simulink model "PID_Controller"  (R2018b)
settings: Solver=ode23s  StartTime=0.0  StopTime=10.0  RelTol=1e-3  AbsTol=AUTO  EnableMultiTasking=on
undefined symbols (not defined in the file or in its folder): Fmatrix, Imatrix
libraries: dspinverses x1
(part 1 of 5)
settings Model: Creator=as01398  LastModifiedBy=jiang
settings SolverCC: MaxConsecutiveMinStep=500
settings DataIOCC: OutputOption=SpecifiedOutputTimes  OutputTimes=[0:0.2:10]
settings OptimizationCC: LifeSpan=inf
settings DebuggingCC: SFUnexpectedBacktrackingDiag=warning  SFNoUnconditionalDefaultTransitionDiag=warning
settings SFSimCC: SimUseLocalCustomCode=off
settings RTWCC: RTWUseLocalCustomCode=off
settings CodeAppCC: StateflowObjectComments=on
settings GRTTargetCC: TargetLangStandard=C89/C90 (ANSI)  GeneratePreprocessorConditionals=Disable all
settings ConfigComp: CovMetricSettings=dw  CovHtmlReporting=on  CovSaveCumulativeToWorkspaceVar=on  CovSaveSingleToWorkspaceVar=on  CovExternalEMLEnable=off

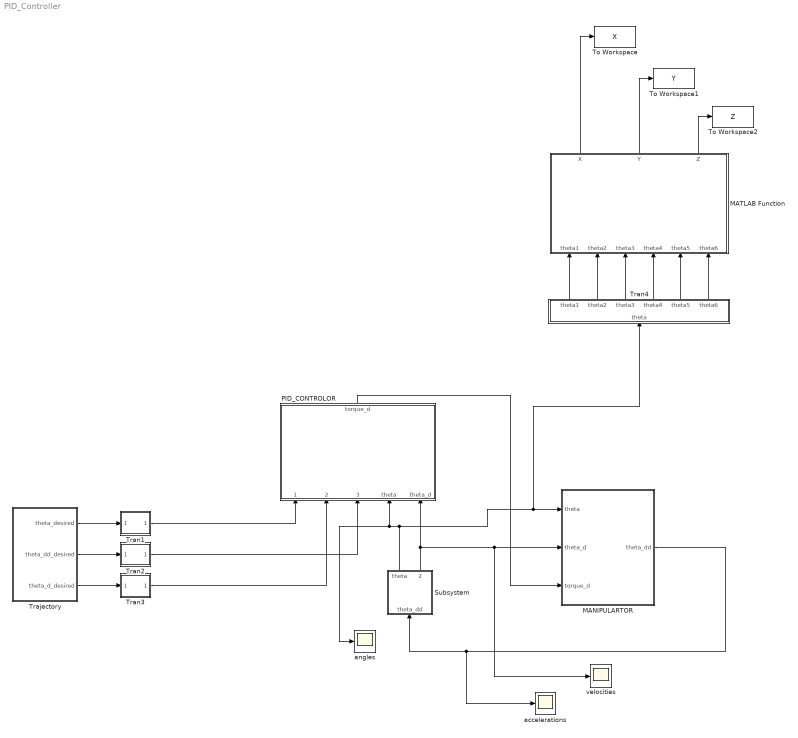
== system PID_Controller ==
  MANIPULARTOR : Subsystem
  MATLAB Function : MATLAB Function  TreatAsAtomicUnit=on
  PID_CONTROLOR : Subsystem
  Subsystem : Subsystem
  To Workspace : ToWorkspace  VariableName=X  SaveFormat=Timeseries  SampleTime=-1
  To Workspace1 : ToWorkspace  VariableName=Y  SaveFormat=Timeseries  SampleTime=-1
  To Workspace2 : ToWorkspace  VariableName=Z  SaveFormat=Timeseries  SampleTime=-1
  Trajectory : Subsystem
  Tran1 : Subsystem
  Tran2 : Subsystem
  Tran3 : Subsystem
  Tran4 : Subsystem
  accelerations : Scope
  angles : Scope
  velocities : Scope
  wires:
  MANIPULARTOR/1(theta_dd) -> accelerations/1, Subsystem/1(theta_dd)
  Subsystem/1(theta) -> PID_CONTROLOR/4(theta), angles/1, Tran4/1(theta), MANIPULARTOR/1(theta)
  Subsystem/2(theta_d) -> PID_CONTROLOR/5(theta_d), velocities/1, MANIPULARTOR/2(theta_d)
  MATLAB Function/1(X) -> To Workspace/1
  MATLAB Function/2(Y) -> To Workspace1/1
  MATLAB Function/3(Z) -> To Workspace2/1
  PID_CONTROLOR/1(torque_d) -> MANIPULARTOR/3(torque_d)
  Trajectory/1(theta_desired) -> Tran1/1(In1)
  Tran1/1(Out2) -> PID_CONTROLOR/1(theta_desired)
  Trajectory/2(theta_dd_desired) -> Tran2/1(In1)
  Tran2/1(Out2) -> PID_CONTROLOR/3(theta_dd_desired)
  Trajectory/3(theta_d_desired) -> Tran3/1(In1)
  Tran3/1(Out2) -> PID_CONTROLOR/2(theta_d_desired)
  Tran4/1(theta1) -> MATLAB Function/1(theta1)
  Tran4/2(theta2) -> MATLAB Function/2(theta2)
  Tran4/3(theta3) -> MATLAB Function/3(theta3)
  Tran4/4(theta4) -> MATLAB Function/4(theta4)
  Tran4/5(theta5) -> MATLAB Function/5(theta5)
  Tran4/6(theta6) -> MATLAB Function/6(theta6)

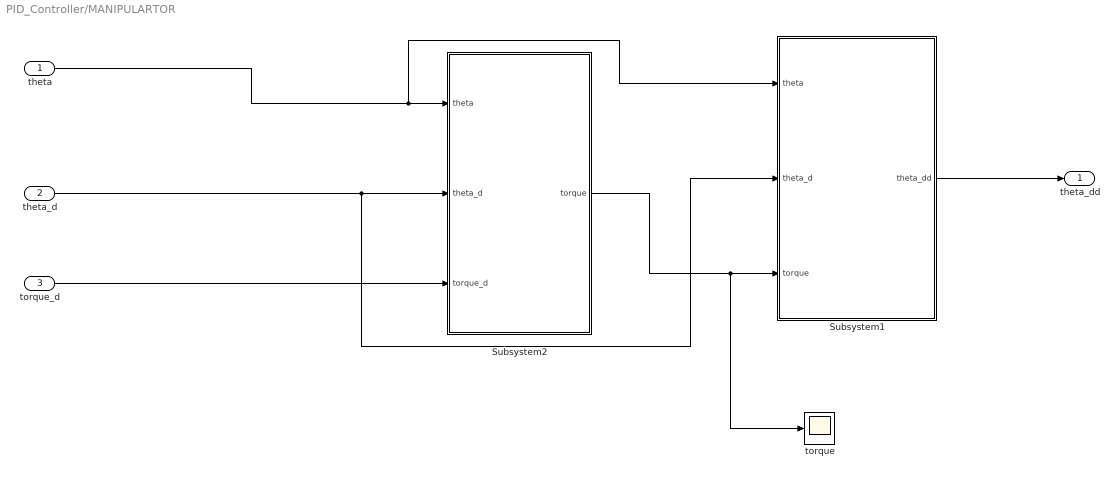
== system PID_Controller/MANIPULARTOR ==
  theta : Inport
  theta_d : Inport  Port=2
  torque_d : Inport  Port=3
  Subsystem1 : Subsystem
  Subsystem2 : Subsystem
  torque : Scope
  theta_dd : Outport
  wires:
  Subsystem1/1(theta_dd) -> theta_dd/1
  torque_d/1 -> Subsystem2/3(torque_d)
  Subsystem2/1(torque) -> torque/1, Subsystem1/3(torque)
  theta/1 -> Subsystem1/1(theta), Subsystem2/1(theta)
  theta_d/1 -> Subsystem1/2(theta_d), Subsystem2/2(theta_d)

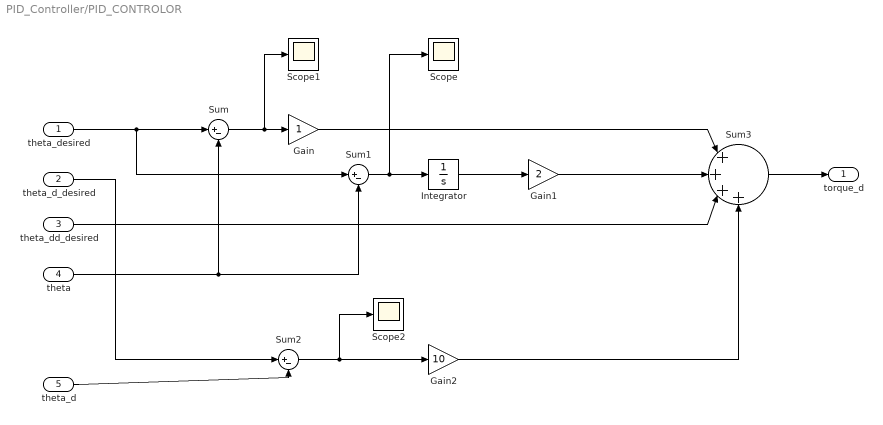
== system PID_Controller/PID_CONTROLOR ==
  theta_desired : Inport
  theta_d_desired : Inport  Port=2
  theta_dd_desired : Inport  Port=3
  theta : Inport  Port=4
  theta_d : Inport  Port=5
  Gain : Gain
  Gain1 : Gain  Gain=2
  Gain2 : Gain  Gain=10
  Integrator : Integrator
  Scope : Scope
  Scope1 : Scope
  Scope2 : Scope
  Sum : Sum  Inputs=|+-
  Sum1 : Sum  Inputs=|+-
  Sum2 : Sum  Inputs=|+-
  Sum3 : Sum  Inputs=|++++
  torque_d : Outport
  wires:
  Sum3/1 -> torque_d/1
  theta_dd_desired/1 -> Sum3/3
  theta_desired/1 -> Sum1/1, Sum/1
  theta/1 -> Sum1/2, Sum/2
  Sum/1 -> Scope1/1, Gain/1
  Sum1/1 -> Integrator/1, Scope/1
  Gain/1 -> Sum3/1
  Gain1/1 -> Sum3/2
  Integrator/1 -> Gain1/1
  Gain2/1 -> Sum3/4
  Sum2/1 -> Scope2/1, Gain2/1
  theta_d_desired/1 -> Sum2/1
  theta_d/1 -> Sum2/2

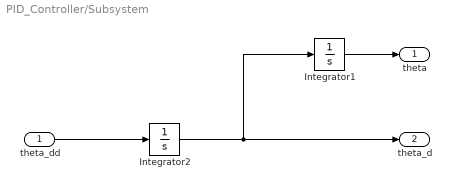
== system PID_Controller/Subsystem ==
  theta_dd : Inport
  Integrator1 : Integrator
  Integrator2 : Integrator
  theta : Outport
  theta_d : Outport  Port=2
  wires:
  theta_dd/1 -> Integrator2/1
  Integrator1/1 -> theta/1
  Integrator2/1 -> theta_d/1, Integrator1/1

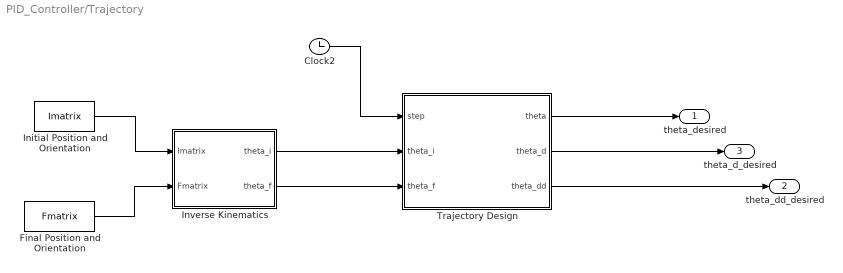
== system PID_Controller/Trajectory ==
  Clock2 : Clock
      settings: Decimation=1000
  Final Position and Orientation : Constant  Value=Fmatrix
  Initial Position and Orientation : Constant  Value=Imatrix
  Inverse Kinematics : MATLAB Function  TreatAsAtomicUnit=on
  Trajectory Design : MATLAB Function  TreatAsAtomicUnit=on
  theta_desired : Outport
  theta_dd_desired : Outport  Port=2
  theta_d_desired : Outport  Port=3
  wires:
  Trajectory Design/3(theta_dd) -> theta_dd_desired/1
  Trajectory Design/2(theta_d) -> theta_d_desired/1
  Trajectory Design/1(theta) -> theta_desired/1
  Inverse Kinematics/2(theta_f) -> Trajectory Design/3(theta_f)
  Inverse Kinematics/1(theta_i) -> Trajectory Design/2(theta_i)
  Final Position and Orientation/1 -> Inverse Kinematics/2(Fmatrix)
  Initial Position and Orientation/1 -> Inverse Kinematics/1(Imatrix)
  Clock2/1 -> Trajectory Design/1(step)

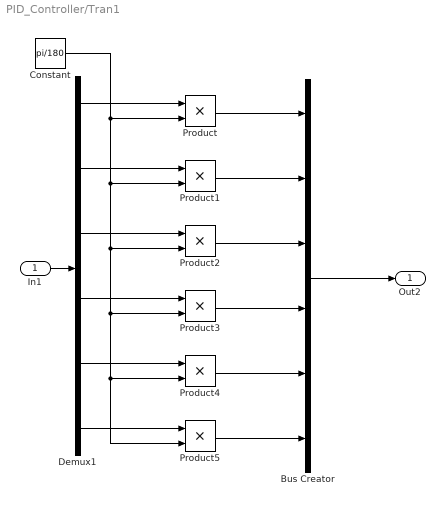
== system PID_Controller/Tran1 ==
  In1 : Inport
  Bus Creator : BusCreator  Inputs=6
  Constant : Constant  Value=pi/180
  Demux1 : Demux  Outputs=6
  Product{,1..5} (6 alike) : Product
  Out2 : Outport
  wires:
  In1/1 -> Demux1/1
  Demux1/1 -> Product/1
  Demux1/2 -> Product1/1
  Demux1/3 -> Product2/1
  Demux1/4 -> Product3/1
  Demux1/5 -> Product4/1
  Demux1/6 -> Product5/1
  Constant/1 -> Product/2, Product1/2, Product2/2, Product3/2, Product5/2, Product4/2
  Product/1 -> Bus Creator/1
  Product1/1 -> Bus Creator/2
  Product2/1 -> Bus Creator/3
  Product3/1 -> Bus Creator/4
  Product4/1 -> Bus Creator/5
  Product5/1 -> Bus Creator/6
  Bus Creator/1 -> Out2/1

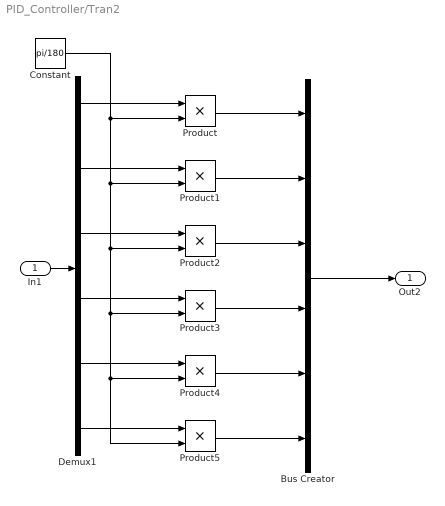
== system PID_Controller/Tran2 ==
  In1 : Inport
  Bus Creator : BusCreator  Inputs=6
  Constant : Constant  Value=pi/180
  Demux1 : Demux  Outputs=6
  Product{,1..5} (6 alike) : Product
  Out2 : Outport
  wires:
  In1/1 -> Demux1/1
  Demux1/1 -> Product/1
  Demux1/2 -> Product1/1
  Demux1/3 -> Product2/1
  Demux1/4 -> Product3/1
  Demux1/5 -> Product4/1
  Demux1/6 -> Product5/1
  Constant/1 -> Product/2, Product1/2, Product2/2, Product3/2, Product5/2, Product4/2
  Product/1 -> Bus Creator/1
  Product1/1 -> Bus Creator/2
  Product2/1 -> Bus Creator/3
  Product3/1 -> Bus Creator/4
  Product4/1 -> Bus Creator/5
  Product5/1 -> Bus Creator/6
  Bus Creator/1 -> Out2/1

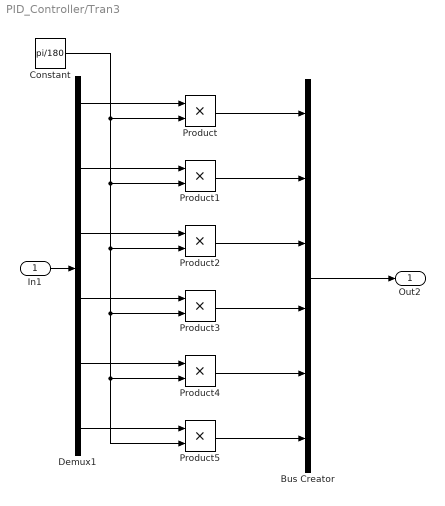
== system PID_Controller/Tran3 ==
  In1 : Inport
  Bus Creator : BusCreator  Inputs=6
  Constant : Constant  Value=pi/180
  Demux1 : Demux  Outputs=6
  Product{,1..5} (6 alike) : Product
  Out2 : Outport
  wires:
  In1/1 -> Demux1/1
  Demux1/1 -> Product/1
  Demux1/2 -> Product1/1
  Demux1/3 -> Product2/1
  Demux1/4 -> Product3/1
  Demux1/5 -> Product4/1
  Demux1/6 -> Product5/1
  Constant/1 -> Product/2, Product1/2, Product2/2, Product3/2, Product5/2, Product4/2
  Product/1 -> Bus Creator/1
  Product1/1 -> Bus Creator/2
  Product2/1 -> Bus Creator/3
  Product3/1 -> Bus Creator/4
  Product4/1 -> Bus Creator/5
  Product5/1 -> Bus Creator/6
  Bus Creator/1 -> Out2/1

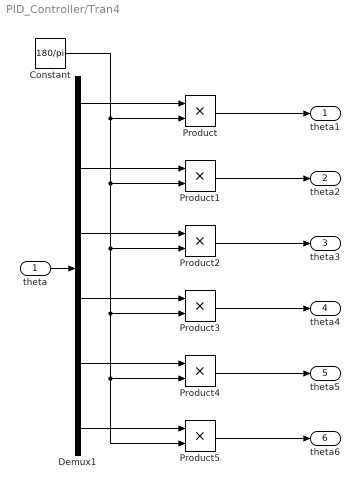
== system PID_Controller/Tran4 ==
  theta : Inport
  Constant : Constant  Value=180/pi
  Demux1 : Demux  Outputs=6
  Product{,1..5} (6 alike) : Product
  theta1 : Outport
  theta2 : Outport  Port=2
  theta3 : Outport  Port=3
  theta4 : Outport  Port=4
  theta5 : Outport  Port=5
  theta6 : Outport  Port=6
  wires:
  theta/1 -> Demux1/1
  Demux1/1 -> Product/1
  Demux1/2 -> Product1/1
  Demux1/3 -> Product2/1
  Demux1/4 -> Product3/1
  Demux1/5 -> Product4/1
  Demux1/6 -> Product5/1
  Constant/1 -> Product/2, Product1/2, Product2/2, Product3/2, Product5/2, Product4/2
  Product/1 -> theta1/1
  Product1/1 -> theta2/1
  Product2/1 -> theta3/1
  Product3/1 -> theta4/1
  Product4/1 -> theta5/1
  Product5/1 -> theta6/1

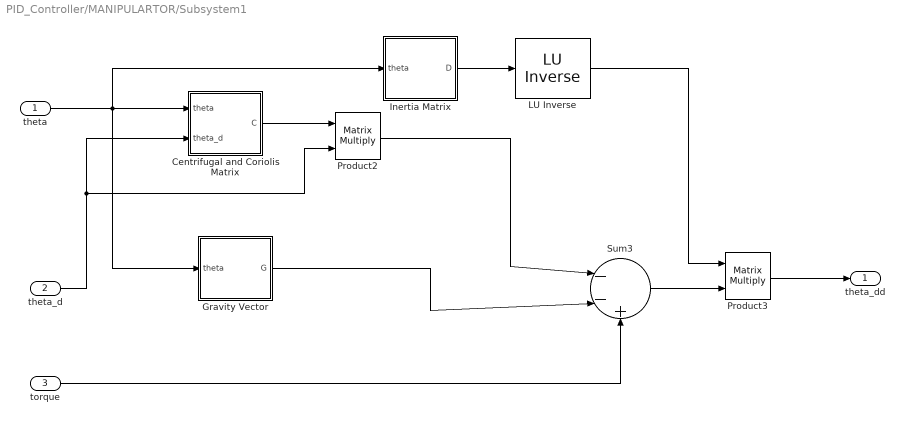
== system PID_Controller/MANIPULARTOR/Subsystem1 ==
  theta : Inport
  theta_d : Inport  Port=2
  torque : Inport  Port=3
  " LU Inverse" : dspinverses/ LU Inverse
      settings: SourceProductName=DSP System Toolbox
  Centrifugal and Coriolis Matrix : Subsystem
  Gravity Vector : Subsystem
  Inertia Matrix : Subsystem
  Product2 : Product  Multiplication=Matrix(*)
  Product3 : Product  Multiplication=Matrix(*)
  Sum3 : Sum  Inputs=|--+
  theta_dd : Outport
  wires:
  Product3/1 -> theta_dd/1
  theta/1 -> Inertia Matrix/1(theta), Gravity Vector/1(theta), Centrifugal and Coriolis Matrix/1(theta)
  theta_d/1 -> Product2/2, Centrifugal and Coriolis Matrix/2(theta_d)
  torque/1 -> Sum3/3
  Gravity Vector/1(G) -> Sum3/2
  Centrifugal and Coriolis Matrix/1(C) -> Product2/1
  Product2/1 -> Sum3/1
  Sum3/1 -> Product3/2
  Inertia Matrix/1(D) -> " LU Inverse"/1
  " LU Inverse"/1 -> Product3/1

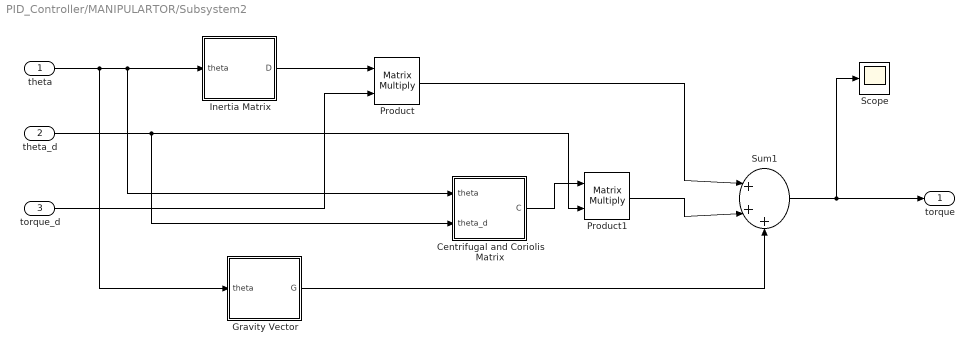
== system PID_Controller/MANIPULARTOR/Subsystem2 ==
  theta : Inport
  theta_d : Inport  Port=2
  torque_d : Inport  Port=3
  Centrifugal and Coriolis Matrix : Subsystem
  Gravity Vector : Subsystem
  Inertia Matrix : Subsystem
  Product : Product  Multiplication=Matrix(*)
  Product1 : Product  Multiplication=Matrix(*)
  Scope : Scope
  Sum1 : Sum  Inputs=|+++
  torque : Outport
  wires:
  theta_d/1 -> Centrifugal and Coriolis Matrix/2(theta_d), Product1/2
  Product/1 -> Sum1/1
  torque_d/1 -> Product/2
  Sum1/1 -> torque/1, Scope/1
  Gravity Vector/1(G) -> Sum1/3
  theta/1 -> Gravity Vector/1(theta), Centrifugal and Coriolis Matrix/1(theta), Inertia Matrix/1(theta)
  Inertia Matrix/1(D) -> Product/1
  Product1/1 -> Sum1/2
  Centrifugal and Coriolis Matrix/1(C) -> Product1/1

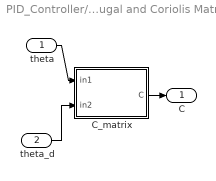
== system PID_Controller/MANIPULARTOR/Subsystem1/Centrifugal and Coriolis Matrix ==
  theta : Inport
  theta_d : Inport  Port=2
  C_matrix : MATLAB Function  TreatAsAtomicUnit=on
  C : Outport
  wires:
  theta_d/1 -> C_matrix/2(in2)
  theta/1 -> C_matrix/1(in1)
  C_matrix/1(C) -> C/1

== system PID_Controller/MANIPULARTOR/Subsystem1/Gravity Vector ==
  theta : Inport
  G_matrix : MATLAB Function  TreatAsAtomicUnit=on
  G : Outport
  wires:
  G_matrix/1(G) -> G/1
  theta/1 -> G_matrix/1(in1)

== system PID_Controller/MANIPULARTOR/Subsystem1/Inertia Matrix ==
  theta : Inport
  D_matrix : MATLAB Function  TreatAsAtomicUnit=on
  D : Outport
  wires:
  D_matrix/1(D) -> D/1
  theta/1 -> D_matrix/1(in1)

== system PID_Controller/MANIPULARTOR/Subsystem2/Centrifugal and Coriolis Matrix ==
  theta : Inport
  theta_d : Inport  Port=2
  C_matrix : MATLAB Function  TreatAsAtomicUnit=on
  C : Outport
  wires:
  theta_d/1 -> C_matrix/2(in2)
  theta/1 -> C_matrix/1(in1)
  C_matrix/1(C) -> C/1

== system PID_Controller/MANIPULARTOR/Subsystem2/Gravity Vector ==
  theta : Inport
  G_matrix : MATLAB Function  TreatAsAtomicUnit=on
  G : Outport
  wires:
  G_matrix/1(G) -> G/1
  theta/1 -> G_matrix/1(in1)

== system PID_Controller/MANIPULARTOR/Subsystem2/Inertia Matrix ==
  theta : Inport
  D_matrix : MATLAB Function  TreatAsAtomicUnit=on
  D : Outport
  wires:
  D_matrix/1(D) -> D/1
  theta/1 -> D_matrix/1(in1)

== matlab function PID_Controller/Trajectory/Inverse Kinematics ==
  data: Imatrix input; theta_i output; theta_f output; Fmatrix input
function [theta_i,theta_f]=IK(Imatrix,Fmatrix)

theta_i=[0;0;0;0;0;0];
theta_f=[0;0;0;0;0;0];
% Initial angles
coder.extrinsic('InverseKinematic')
[qi1,qi2,qi3,qi4,qi5,qi6]=InverseKinematic(Imatrix);
    q01=qi1;
    q02=qi2;
    q03=qi3;
    q04=qi4;
    q05=qi5;
    q06=qi6;
    
% Final angles
[qi1,qi2,qi3,qi4,qi5,qi6]=InverseKinematic(Fmatrix);
    qf1=qi1;
    qf2=qi2;
    qf3=qi3;
    qf4=qi4;
    qf5=qi5;
    qf6=qi6;

theta_i=[q01;q02;q03;q04;q05;q06];
theta_f=[qf1;qf2;qf3;qf4;qf5;qf6];

== matlab function PID_Controller/MANIPULARTOR/Subsystem1/Inertia Matrix/D_matrix ==
  data: in1 input; D output
function D = Dmatrix(in1)

D=zeros(6,6);
%DMATRIX
%    D = DMATRIX(IN1)

%    This function was generated by the Symbolic Math Toolbox version 7.0.
%    08-Aug-2017 16:41:29

q1 = in1(1,:);
q2 = in1(2,:);
q3 = in1(3,:);
q4 = in1(4,:);
q5 = in1(5,:);
q6 = in1(6,:);
t2 = cos(q1);
t3 = cos(q6);
t4 = sin(q6);
t5 = sin(q1);
t6 = cos(q2);
t7 = sin(q2);
t8 = cos(q4);
t9 = sin(q4);
t10 = t2.*t4.*(2.0./1.25e2);
t72 = t3.*t5.*(2.0./1.25e2);
t11 = t10-t72;
t12 = t2.*t3.*(2.0./1.25e2);
t13 = t4.*t5.*(2.0./1.25e2);
t14 = t12+t13;
t15 = t2.*t7.*(7.0./2.0e2);
t77 = t5.*t6.*(7.0./2.0e2);
t16 = t15-t77;
t17 = t2.*t6.*(3.0./2.0e2);
t18 = t5.*t7.*(3.0./2.0e2);
t19 = t17+t18;
t20 = t2.*t9.*(1.0./2.0e2);
t82 = t5.*t8.*(1.0./2.0e2);
t21 = t20-t82;
t22 = t2.*t8.*(3.0./1.0e3);
t23 = t5.*t9.*(3.0./1.0e3);
t24 = t22+t23;
t25 = cos(q3);
t26 = sin(q3);
t27 = t2.*t6.*t26;
t28 = t2.*t7.*t25;
t29 = t27+t28;
t30 = t6.*t25;
t59 = t7.*t26;
t31 = t30-t59;
t32 = t5.*(1.0./4.0);
t38 = t2.*t6.*(1.0./2.0);
t33 = t32-t38;
t34 = sin(q5);
t35 = cos(q5);
t36 = t5.*t6.*t26;
t37 = t5.*t7.*t25;
t39 = t5.*t9;
t40 = t2.*t6.*t25;
t67 = t2.*t7.*t26;
t41 = t40-t67;
t68 = t8.*t41;
t42 = t39-t68;
t43 = t29.*t35;
t44 = t2.*(1.0./4.0);
t45 = t5.*t6.*(1.0./2.0);
t46 = t36+t37+t44+t45;
t69 = t34.*t42;
t47 = t43-t69;
t48 = t2.*t9;
t49 = t5.*t6.*t25;
t58 = t5.*t7.*t26;
t135 = t49-t58;
t50 = t8.*t135;
t51 = t48+t50;
t52 = t34.*t51;
t53 = t36+t37;
t54 = t35.*t53;
t55 = t52+t54;
t56 = t27+t28-t32+t38;
t57 = t44+t45;
t60 = t7.*(1.0./2.0);
t61 = -t30+t59+t60;
t62 = t31.*t35;
t63 = t6.*t26;
t64 = t7.*t25;
t65 = t63+t64;
t70 = t8.*t34.*t65;
t66 = t62-t70;
t71 = t3.*t14;
t73 = t4.*t11;
t74 = t71+t73;
t75 = t2.*t74;
t76 = t6.*t19;
t78 = t7.*t16;
t79 = t76+t78;
t80 = t2.*t79;
t81 = t8.*t24;
t83 = t9.*t21;
t84 = t81+t83;
t85 = t2.*t84;
t86 = t3.*t11;
t128 = t4.*t14;
t87 = t86-t128;
t88 = t6.*t16;
t162 = t7.*t19;
t89 = t88-t162;
t90 = t8.*t21;
t129 = t9.*t24;
t91 = t90-t129;
t92 = t7.*t29.*(1.0./2.0);
t165 = t31.*t33;
t93 = t92-t165;
t94 = t7.*t29.*(8.0./5.0);
t140 = t31.*t33.*(1.6e1./5.0);
t95 = t94-t140;
t96 = t93.*t95;
t97 = t46.*t47;
t98 = t46.*t47.*(1.0./2.0);
t130 = t55.*t56.*(1.0./2.0);
t131 = t98-t130;
t99 = t131.*(t97-t55.*t56);
t100 = t29.*t57;
t101 = t33.*t53;
t102 = t100+t101;
t103 = t29.*t57.*(1.6e1./5.0);
t104 = t33.*t53.*(1.6e1./5.0);
t105 = t103+t104;
t106 = t102.*t105;
t107 = t55.*t61;
t108 = t46.*t66;
t109 = t107+t108;
t110 = t55.*t61.*(1.0./2.0);
t111 = t46.*t66.*(1.0./2.0);
t112 = t110+t111;
t113 = t109.*t112;
t114 = t31.*t57;
t115 = t7.*t53.*(1.0./2.0);
t116 = t114+t115;
t117 = t31.*t57.*(1.6e1./5.0);
t118 = t7.*t53.*(8.0./5.0);
t119 = t117+t118;
t120 = t116.*t119;
t121 = t47.*t61;
t122 = t56.*t66;
t123 = t47.*t61.*(1.0./2.0);
t124 = t56.*t66.*(1.0./2.0);
t127 = t123+t124;
t212 = t121+t122;
t125 = t127.*t212;
t161 = t5.*t87;
t163 = t5.*t89;
t164 = t5.*t91;
t126 = t75+t80+t85+t96+t99+t106+t113+t120+t125-t161-t163-t164;
t132 = t5.*t8;
t133 = t9.*t41;
t134 = t132+t133;
t136 = t2.*t8;
t183 = t9.*t135;
t137 = t136-t183;
t138 = t31.*t47;
t175 = t29.*t66;
t139 = t138-t175;
t141 = t5.*t8.*(1.09e2./1.0e3);
t142 = t9.*t41.*(1.09e2./1.0e3);
t143 = -t32+t38+t141+t142;
t186 = t9.*t65.*(1.09e2./1.0e3);
t144 = t60-t186;
t145 = t9.*(t49-t58).*(1.09e2./1.0e3);
t190 = t2.*t8.*(1.09e2./1.0e3);
t146 = t44+t45+t145-t190;
t147 = t8.*(t49-t58);
t148 = t48+t147;
t149 = t34.*t148;
t150 = t54+t149;
t151 = t87.*(t43-t69);
t152 = t74.*t150;
t153 = t61.*t150.*(1.0./2.0);
t154 = t111+t153;
t199 = t34.*t148.*(1.1e1./5.0e2);
t200 = t35.*t53.*(1.1e1./5.0e2);
t155 = t36+t37+t44+t45-t199-t200;
t166 = t56.*t150.*(1.0./2.0);
t156 = t98-t166;
t157 = t34.*t42.*(1.1e1./5.0e2);
t205 = t29.*t35.*(1.1e1./5.0e2);
t158 = t27+t28-t32+t38+t157-t205;
t159 = t8.*t34.*t65.*(1.1e1./5.0e2);
t202 = t31.*t35.*(1.1e1./5.0e2);
t160 = -t30+t59+t60+t159-t202;
t167 = t2.^2;
t168 = t5.^2;
t213 = t56.*t150;
t169 = (t98-t166).*(t97-t213);
t170 = t61.*t150;
t171 = t108+t170;
t172 = t154.*t171;
t173 = t6.^2;
t174 = (t121+t122).*(t123+t124);
t176 = t29.*t87;
t177 = t29.*t91;
t178 = t53.*t74;
t179 = t53.*t84;
t180 = t47.*t53;
t181 = t53.*t66;
t197 = t31.*t150;
t349 = t181-t197;
t182 = t154.*t349;
t184 = t74.*t137;
t185 = t84.*t137;
t187 = t29.*t144;
t188 = t31.*t143;
t189 = t187+t188;
t191 = t29.*t146;
t301 = t53.*t143;
t192 = t191-t301;
t193 = t53.*t144;
t194 = t31.*t146;
t195 = t193+t194;
t243 = t29.*t150;
t196 = (t98-t166).*(t180-t243);
t198 = t151+t152;
t201 = t66.*t155;
t203 = t150.*t160;
t204 = t201+t203;
t206 = t47.*t155;
t260 = t150.*t158;
t207 = t206-t260;
t208 = t66.*t158;
t209 = t47.*t160;
t210 = t208+t209;
t211 = t151+t152-t127.*t210-t154.*t204-t156.*t207;
t214 = t3.*t29.*(2.0./1.25e2);
t215 = t4.*t53.*(2.0./1.25e2);
t216 = t214+t215;
t217 = t4.*t29.*(2.0./1.25e2);
t228 = t3.*t53.*(2.0./1.25e2);
t218 = t217-t228;
t219 = t8.*t29.*(1.0./2.0e2);
t220 = t9.*t53.*(1.0./2.0e2);
t221 = t219+t220;
t222 = t9.*t29.*(3.0./1.0e3);
t231 = t8.*t53.*(3.0./1.0e3);
t223 = t222-t231;
t224 = t31.*t47.*(1.0./2.0);
t248 = t29.*t66.*(1.0./2.0);
t225 = t224-t248;
t226 = t47.*t53.*(1.0./2.0);
t244 = t29.*t150.*(1.0./2.0);
t261 = t226-t244;
t227 = t261.*(t97-t213);
t229 = t4.*t216;
t245 = t3.*t218;
t230 = t2.*(t229-t245);
t232 = t9.*t221;
t246 = t8.*t223;
t233 = t2.*(t232-t246);
t234 = t3.*t216;
t235 = t4.*t218;
t236 = t234+t235;
t237 = t8.*t221;
t238 = t9.*t223;
t239 = t237+t238;
t240 = t53.*t66.*(1.0./2.0);
t247 = t31.*t150.*(1.0./2.0);
t259 = t240-t247;
t241 = t171.*t259;
t263 = t212.*t225;
t242 = t227+t230+t233+t241-t263-t5.*t236-t5.*t239;
t249 = (t180-t243).*(t226-t244);
t250 = (t181-t197).*(t240-t247);
t251 = (t138-t175).*(t224-t248);
t252 = t6.*t25.*(1.0./1.25e2);
t256 = t7.*t26.*(1.0./1.25e2);
t253 = t252-t256;
t254 = t6.*t25.*(1.0./2.5e2);
t255 = t254-t7.*t26.*(1.0./2.5e2);
t257 = t236.*(t43-t69);
t258 = t150.*(t229-t245);
t262 = t66.*t253;
t264 = t3.*t134.*(2.0./1.25e2);
t279 = t4.*t137.*(2.0./1.25e2);
t265 = t264-t279;
t266 = t3.*t137.*(2.0./1.25e2);
t267 = t4.*t134.*(2.0./1.25e2);
t268 = t266+t267;
t269 = t8.*t134.*(1.0./2.0e2);
t282 = t9.*t137.*(1.0./2.0e2);
t270 = t269-t282;
t271 = t8.*t137.*(3.0./1.0e3);
t272 = t9.*t134.*(3.0./1.0e3);
t273 = t271+t272;
t274 = t29.*t144.*(1.6e1./5.0);
t275 = t31.*t143.*(1.6e1./5.0);
t276 = t274+t275;
t277 = t29.*t146.*(1.6e1./5.0);
t302 = t53.*t143.*(1.6e1./5.0);
t278 = t277-t302;
t280 = t4.*t265;
t299 = t3.*t268;
t281 = t280-t299;
t283 = t9.*t270;
t300 = t8.*t273;
t284 = t283-t300;
t285 = t3.*t265;
t286 = t4.*t268;
t287 = t285+t286;
t288 = t5.*t287;
t289 = t8.*t270;
t290 = t9.*t273;
t291 = t289+t290;
t292 = t5.*t291;
t293 = t53.*t144.*(1.6e1./5.0);
t294 = t31.*t146.*(1.6e1./5.0);
t295 = t293+t294;
t296 = (t97-t213).*(t226-t244);
t297 = t171.*(t240-t247);
t298 = -t263+t288+t292+t296+t297-t2.*t281-t2.*t284-t93.*t276-t102.*t278-t116.*t295;
t303 = t160.*(t43-t69);
t304 = t208+t303;
t305 = t304.*(t224-t248);
t306 = t9.*t65.*t66.*(1.0./1.25e2);
t307 = t3.*t47.*(2.0./1.25e2);
t308 = t4.*t150.*(2.0./1.25e2);
t309 = t307+t308;
t310 = t4.*t47.*(2.0./1.25e2);
t312 = t3.*t150.*(2.0./1.25e2);
t311 = t310-t312;
t313 = t3.*t309;
t314 = t4.*t311;
t315 = t313+t314;
t316 = t4.*(t307+t308);
t318 = t3.*t311;
t317 = t316-t318;
t319 = t31.*t35.*(1.0./1.25e2);
t324 = t8.*t34.*t65.*(1.0./1.25e2);
t320 = t319-t324;
t321 = -t43+t69;
t322 = t4.*t321.*(2.0./1.25e2);
t323 = t312+t322;
t330 = t3.*t321.*(2.0./1.25e2);
t325 = t308-t330;
t326 = t4.*t323;
t334 = t3.*t325;
t327 = t326-t334;
t328 = t321.*t327;
t329 = t3.*t323;
t331 = t66.*t320;
t332 = t4.*(t308-t330);
t333 = t329+t332;
t335 = t2.*t333;
t336 = t5.*t327;
t337 = t66.*t155.*(1.0./2.0);
t338 = t150.*t160.*(1.0./2.0);
t339 = t337+t338;
t340 = t46.*t321;
t341 = t213+t340;
t342 = t150.*t158.*(1.0./2.0);
t343 = t155.*t321.*(1.0./2.0);
t344 = t342+t343;
t345 = t66.*t158.*(1.0./2.0);
t350 = t160.*t321.*(1.0./2.0);
t346 = t345-t350;
t347 = t122-t61.*t321;
t348 = t335+t336-t171.*t339-t341.*t344-t346.*t347;
t351 = t31.*t320;
t352 = t53.*t321;
t353 = t243+t352;
t354 = t31.*t321;
t355 = t175+t354;
t356 = t9.*t65.*t320;
t357 = t150.*t333;
t358 = t328+t331+t357;
D = reshape([t126,t75+t80+t85+t96+t106+t120-t161-t163-t164+t169+t172+t174,t242,t298,-t5.*t315+t2.*(t4.*t309-t3.*t311),t348,t126,t75+t80+t85+t96+t106+t120-t161-t163-t164+t169+t172+t174+(t7.*t167.*(3.3e1./2.5e2)+t7.*t168.*(3.3e1./2.5e2)).*(t7.*t167.*(2.97e2./6.25e2)+t7.*t168.*(2.97e2./6.25e2))+t167.*t173.*6.27264e-2+t168.*t173.*6.27264e-2,t242,t298,t2.*t317-t5.*t315,t348,t176+t177+t178+t179-t127.*t139-t131.*(t29.*t55-t47.*t53)-t112.*(t31.*t55-t53.*t66),t176+t177+t178+t179+t182+t196-t127.*t139,t249+t250+t251+t29.*t236+t29.*t239+t31.*t253+t31.*t255+t53.*(t229-t245)+t53.*(t232-t246),t249+t250+t251-t29.*t287-t29.*t291-t53.*t281-t53.*t284+t9.*t31.*t65.*(3.0./2.5e2),t351+t29.*(t313+t314)+t53.*t317,t351-t29.*t327+t53.*t333-t339.*t349-t344.*t353-t346.*t355,t182+t184+t185-t87.*t134-t91.*t134-t127.*t139-t95.*t189-t105.*t192-t119.*t195+t156.*(t180-t29.*t150),t182+t184+t185+t196-t87.*t134-t91.*t134-t127.*t139-t95.*t189-t105.*t192-t119.*t195,t249+t250+t251-t134.*t236-t134.*t239+t137.*(t229-t245)+t137.*(t232-t246)+t9.*t65.*t253+t9.*t65.*t255,t249+t250+t251+t9.^2.*t65.^2.*(3.0./2.5e2)-t137.*t281+t134.*t287-t137.*t284+t134.*t291+t189.*t276+t192.*t278+t195.*t295,t356-t134.*t315+t137.*t317,t356+t134.*t327+t137.*t333-t339.*t349-t344.*t353-t346.*t355,t198,t198,t257+t258+t262,t306-t47.*t287-t150.*t281,t328+t331+t150.*(t329+t4.*t325),t358,t211,t211,t257+t258+t262+t305-t204.*t259-t207.*t261,t305+t306-t47.*t287-t150.*t281-t204.*t259-t207.*t261,t358,t328+t331+t357+t204.*t339+t346.*(t208-t160.*t321)+t344.*(t260+t155.*t321)],[6,6]);
